simulink model "NoDCDCConverterSSC"  (R2026b)
settings: Solver=VariableStepAuto
undefined symbols (not defined in the file): EnvAirTemp
libraries: fl_lib x3, nesl_utility x2
settings Model: ModifiedByFormat=The MathWorks, Inc.  Creator=The MathWorks, Inc.  LastModifiedBy=The MathWorks, Inc.
settings OptimizationCC: ReuseModelBlockBuffer=off
settings SimscapeCC: SimscapeUseEnergyAccounting=off

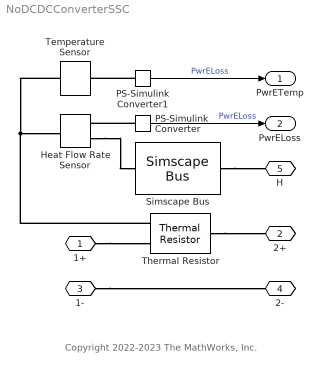
== system NoDCDCConverterSSC ==
  note: Copyright 2022-2023 The MathWorks, Inc.
  Heat Flow Rate Sensor : fl_lib/Thermal/Thermal Sensors/Heat Flow Rate Sensor
  PS-Simulink Converter : nesl_utility/PS-Simulink Converter  PhysicalDomain=network_engine_domain  SubClassName=ps_output  LeftPortType=input  RightPortType=output  PseudoPeriodic=off  Frequencies=[]  VectorFormat=inherit  Unit=inherit  AffineConversion=off
  PS-Simulink Converter1 : nesl_utility/PS-Simulink Converter  PhysicalDomain=network_engine_domain  SubClassName=ps_output  LeftPortType=input  RightPortType=output  PseudoPeriodic=off  Frequencies=[]  VectorFormat=inherit  Unit=inherit  AffineConversion=off
  Simscape Bus : SimscapeBus  HierarchyStrings=ThrmPwrE1
  Temperature Sensor : fl_lib/Thermal/Thermal Sensors/Temperature Sensor  temperature_measure=foundation.enum.MeasurementReference.absolute
  Thermal Resistor : fl_lib/Electrical/Electrical Elements/Thermal Resistor  R0=1e-6 Ohm  T0=EnvAirTemp K  alpha=50e-6 1/K  thermalMassParameterization=foundation.enum.ThermalMassParameterization.TimeConstantAndDissipationFactor  mass=2.6316e-5 kg  cp=380 J/(K*kg)  tc=10 s  K_d=1 W/K  T_specify=on  T_priority=High  T=EnvAirTemp K  T_nominal_specify=off  T_nominal_value=1  T_nominal_unit=K
  1+ : PMIOPort  Side=Left
  2+ : PMIOPort  Port=2  Side=Right
  1- : PMIOPort  Port=3  Side=Left
  2- : PMIOPort  Port=4  Side=Right
  H : PMIOPort  Port=5  Side=Right
  PwrETemp : Outport
  PwrELoss : Outport  Port=2
  wires:
  PS-Simulink Converter/1 -> PwrELoss/1  "PwrELoss"
  PS-Simulink Converter1/1 -> PwrETemp/1  "PwrELoss"
  connections:
  1-/RConn1 -- 2-/RConn1
  Simscape Bus/RConn1 -- H/RConn1
  Thermal Resistor/RConn1 -- 2+/RConn1
  1+/RConn1 -- Thermal Resistor/LConn2
  Heat Flow Rate Sensor/RConn2 -- Simscape Bus/LConn1
  Thermal Resistor/LConn1 -- Temperature Sensor/LConn1 -- Heat Flow Rate Sensor/LConn1
  PS-Simulink Converter/LConn1 -- Heat Flow Rate Sensor/RConn1
  PS-Simulink Converter1/LConn1 -- Temperature Sensor/RConn1
